simulink model "lab20"  (Simulink 7.9)
settings: Solver=ode45  StartTime=0.0  StopTime=10.0  RelTol=1e-3
settings Model: Creator=Mihail  LastModifiedBy=Mihail

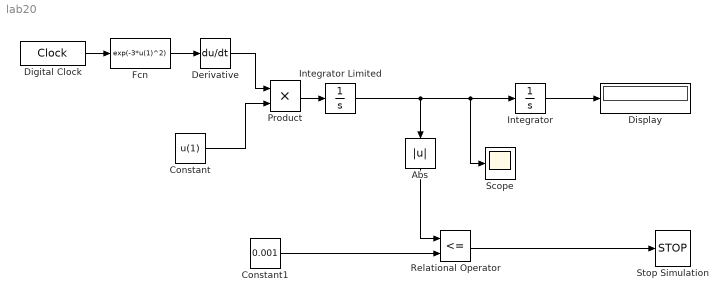
== system lab20 ==
  Abs : Abs
  Constant : Constant  Value=u(1)
  Constant1 : Constant  Value=0.001
  Derivative : Derivative
  Digital Clock : DigitalClock
  Display : Display
  Fcn : Fcn  Expr=exp(-3*u(1)^2)
  Integrator : Integrator
  Integrator Limited : Integrator  LimitOutput=on  UpperSaturationLimit=0.2  LowerSaturationLimit=0
  Product : Product  RndMeth=Zero
  Relational Operator : RelationalOperator  Operator=<=  OutDataTypeStr=boolean
  Scope : Scope
  Stop Simulation : Stop
  wires:
  Integrator/1 -> Display/1
  Constant1/1 -> Relational Operator/2
  Abs/1 -> Relational Operator/1
  Relational Operator/1 -> Stop Simulation/1
  Integrator Limited/1 -> Abs/1, Integrator/1, Scope/1
  Digital Clock/1 -> Fcn/1
  Fcn/1 -> Derivative/1
  Derivative/1 -> Product/1
  Constant/1 -> Product/2
  Product/1 -> Integrator Limited/1
